simulink model "IEEE9Buses"  (R2024b)
settings: Solver=FixedStepAuto  StartTime=0  StopTime=5  FixedStep=1e-6  RelTol=1e-3
values from neighbouring files (symbols this model uses):
  SG_D_1_D = 0.01056    [SG9_parameters.m]
  SG_D_1_EnableSaturation = 0    [SG9_parameters.m]
  SG_D_1_f0 = 60    [SG9_parameters.m]
  SG_D_1_H = 7.5    [SG9_parameters.m]
  SG_D_1_K_A = 20    [SG9_parameters.m]
  SG_D_1_K_E = 1.000000e+1    (= 10)    [SG9_parameters.m]
  SG_D_1_K_F = 2.363    [SG9_parameters.m]
  SG_D_1_K_s = 5    [SG9_parameters.m]
  SG_D_1_R_a = 0.001088    [SG9_parameters.m]
  SG_D_1_S_A = 1    [SG9_parameters.m]
  SG_D_1_S_B = 0.103    [SG9_parameters.m]
  SG_D_1_S_N = 10.659857    [SG9_parameters.m]
  SG_D_1_SpeedPara = 200    [SG9_parameters.m]
  SG_D_1_T_0 = 0.720173    [SG9_parameters.m]
  SG_D_1_T_1 = 0.3    [SG9_parameters.m]
  SG_D_1_T_2 = 0.05    [SG9_parameters.m]
  SG_D_1_T_3 = 0.02    [SG9_parameters.m]
  SG_D_1_T_4 = 0.005    [SG9_parameters.m]
  SG_D_1_T_A = 0.02    [SG9_parameters.m]
  SG_D_1_T_dd = 8.000000e+0    (= 8)    [SG9_parameters.m]
  SG_D_1_T_ddd = 0.04    [SG9_parameters.m]
  SG_D_1_T_E = 0.314    [SG9_parameters.m]
  SG_D_1_T_F = 0.35    [SG9_parameters.m]
  SG_D_1_T_qd = 0.8    [SG9_parameters.m]
  SG_D_1_T_qdd = 0.02    [SG9_parameters.m]
  SG_D_1_T_speed = 0.1    [SG9_parameters.m]
  SG_D_1_T_w = 0.5    [SG9_parameters.m]
  SG_D_1_V_ref = 1.990276    [SG9_parameters.m]
  SG_D_1_w_ref = 376.991118    [SG9_parameters.m]
  SG_D_1_x_d = 1.9    [SG9_parameters.m]
  SG_D_1_x_dd = 0.302    [SG9_parameters.m]
  SG_D_1_x_ddd = 0.204    [SG9_parameters.m]
  SG_D_1_x_l = 0.05    [SG9_parameters.m]
  SG_D_1_x_q = 1.3    [SG9_parameters.m]
  SG_D_1_x_qd = 0.5    [SG9_parameters.m]
  SG_D_1_x_qdd = 0.3    [SG9_parameters.m]
  SG_D_2_D = 0.01056    [SG9_parameters.m]
  SG_D_2_EnableSaturation = 0    [SG9_parameters.m]
  SG_D_2_f0 = 60    [SG9_parameters.m]
  SG_D_2_H = 7.5    [SG9_parameters.m]
  SG_D_2_K_A = 20    [SG9_parameters.m]
  SG_D_2_K_E = 1.000000e+1    (= 10)    [SG9_parameters.m]
  SG_D_2_K_F = 2.363    [SG9_parameters.m]
  SG_D_2_K_s = 0.5    [SG9_parameters.m]
  SG_D_2_R_a = 0.001088    [SG9_parameters.m]
  SG_D_2_S_A = 1    [SG9_parameters.m]
  SG_D_2_S_B = 0.103    [SG9_parameters.m]
  SG_D_2_S_N = 10.659857    [SG9_parameters.m]
  SG_D_2_SpeedPara = 200    [SG9_parameters.m]
  SG_D_2_T_0 = 1.632913    [SG9_parameters.m]
  SG_D_2_T_1 = 0.2    [SG9_parameters.m]
  SG_D_2_T_2 = 0.05    [SG9_parameters.m]
  SG_D_2_T_3 = 0.02    [SG9_parameters.m]
  SG_D_2_T_4 = 0.005    [SG9_parameters.m]
  SG_D_2_T_A = 0.02    [SG9_parameters.m]
  SG_D_2_T_dd = 8.000000e+0    (= 8)    [SG9_parameters.m]
  SG_D_2_T_ddd = 0.04    [SG9_parameters.m]
  SG_D_2_T_E = 0.314    [SG9_parameters.m]
  SG_D_2_T_F = 0.35    [SG9_parameters.m]
  SG_D_2_T_qd = 0.8    [SG9_parameters.m]
  SG_D_2_T_qdd = 0.02    [SG9_parameters.m]
  SG_D_2_T_speed = 0.1    [SG9_parameters.m]
  SG_D_2_T_w = 0.5    [SG9_parameters.m]
  SG_D_2_V_ref = 2.662631    [SG9_parameters.m]
  SG_D_2_w_ref = 376.991118    [SG9_parameters.m]
  SG_D_2_x_d = 1.9    [SG9_parameters.m]
  SG_D_2_x_dd = 0.302    [SG9_parameters.m]
  SG_D_2_x_ddd = 0.204    [SG9_parameters.m]
  SG_D_2_x_l = 0.05    [SG9_parameters.m]
  SG_D_2_x_q = 1.3    [SG9_parameters.m]
  SG_D_2_x_qd = 0.5    [SG9_parameters.m]
  SG_D_2_x_qdd = 0.3    [SG9_parameters.m]
  SG_D_3_D = 0.01056    [SG9_parameters.m]
  SG_D_3_EnableSaturation = 0    [SG9_parameters.m]
  SG_D_3_f0 = 60    [SG9_parameters.m]
  SG_D_3_H = 7.5    [SG9_parameters.m]
  SG_D_3_K_A = 20    [SG9_parameters.m]
  SG_D_3_K_E = 1.000000e+1    (= 10)    [SG9_parameters.m]
  SG_D_3_K_F = 2.363    [SG9_parameters.m]
  SG_D_3_K_s = 0.5    [SG9_parameters.m]
  SG_D_3_R_a = 0.001088    [SG9_parameters.m]
  SG_D_3_S_A = 1    [SG9_parameters.m]
  SG_D_3_S_B = 0.103    [SG9_parameters.m]
  SG_D_3_S_N = 10.659857    [SG9_parameters.m]
  SG_D_3_SpeedPara = 200    [SG9_parameters.m]
  SG_D_3_T_0 = 0.850788    [SG9_parameters.m]
  SG_D_3_T_1 = 0.2    [SG9_parameters.m]
  SG_D_3_T_2 = 0.05    [SG9_parameters.m]
  SG_D_3_T_3 = 0.02    [SG9_parameters.m]
  SG_D_3_T_4 = 0.005    [SG9_parameters.m]
  SG_D_3_T_A = 0.02    [SG9_parameters.m]
  SG_D_3_T_dd = 8.000000e+0    (= 8)    [SG9_parameters.m]
  SG_D_3_T_ddd = 0.04    [SG9_parameters.m]
  SG_D_3_T_E = 0.314    [SG9_parameters.m]
  SG_D_3_T_F = 0.35    [SG9_parameters.m]
  SG_D_3_T_qd = 0.8    [SG9_parameters.m]
  SG_D_3_T_qdd = 0.02    [SG9_parameters.m]
  SG_D_3_T_speed = 0.1    [SG9_parameters.m]
  SG_D_3_T_w = 0.5    [SG9_parameters.m]
  SG_D_3_V_ref = 1.915682    [SG9_parameters.m]
  SG_D_3_w_ref = 376.991118    [SG9_parameters.m]
  SG_D_3_x_d = 1.9    [SG9_parameters.m]
  SG_D_3_x_dd = 0.302    [SG9_parameters.m]
  SG_D_3_x_ddd = 0.204    [SG9_parameters.m]
  SG_D_3_x_l = 0.05    [SG9_parameters.m]
  SG_D_3_x_q = 1.3    [SG9_parameters.m]
  SG_D_3_x_qd = 0.5    [SG9_parameters.m]
  SG_D_3_x_qdd = 0.3    [SG9_parameters.m]
(part 2 of 9)

== system IEEE9Buses/SG_D_3 ==
  v_d_SG_D_3 : Inport
  v_q_SG_D_3 : Inport  Port=2
  E_fd_SG_D_3 : Integrator  InitialCondition=1.8313641649557557
  Px_1_SG_D_3 : Integrator  InitialCondition=0.0
  Px_2_SG_D_3 : Integrator  InitialCondition=0.0
  Px_3_SG_D_3 : Integrator  InitialCondition=2.300913107602939e-24
  R_f_SG_D_3 : Integrator  InitialCondition=12.364324347972719
  T_e_SG_D_3_block : Subsystem
  T_m_SG_D_3 : Integrator  InitialCondition=0.8507875286404913
  V_f_SG_D_3 : Integrator  InitialCondition=18.313641649557557
  d_E_fd_SG_D_3_block : Subsystem
  d_Px_1_SG_D_3_block : Subsystem
  d_Px_2_SG_D_3_block : Subsystem
  d_Px_3_SG_D_3_block : Subsystem
  d_R_f_SG_D_3_block : Subsystem
  d_T_m_SG_D_3_block : Subsystem
  d_V_f_SG_D_3_block : Subsystem
  d_psi_1d_SG_D_3_block : Subsystem
  d_psi_d_SG_D_3_block : Subsystem
  d_psi_fd_SG_D_3_block : Subsystem
  d_psi_gq_SG_D_3_block : Subsystem
  d_psi_kq_SG_D_3_block : Subsystem
  d_psi_q_SG_D_3_block : Subsystem
  d_theta_SG_D_3_block : Subsystem
  d_w_SG_D_3_block : Subsystem
  i_d_SG_D_3_block : Subsystem
  i_q_SG_D_3_block : Subsystem
  psi_1d_SG_D_3 : Integrator  InitialCondition=0.6849000717806094
  psi_d_SG_D_3 : Integrator  InitialCondition=0.6539145557488486
  psi_fd_SG_D_3 : Integrator  InitialCondition=0.8410670725806834
  psi_gq_SG_D_3 : Integrator  InitialCondition=0.46633252147547377
  psi_kq_SG_D_3 : Integrator  InitialCondition=-0.7286445648054278
  psi_q_SG_D_3 : Integrator  InitialCondition=-0.757790347397645
  theta_SG_D_3 : Integrator  InitialCondition=0.9421581999064681
  theta_SG_D_3_out_block : Subsystem
  w_SG_D_3 : Integrator  InitialCondition=376.99111843077515
  w_SG_D_3_out_block : Subsystem
  i_d_SG_D_3 : Outport
  i_q_SG_D_3 : Outport  Port=2
  T_e_SG_D_3 : Outport  Port=3
  w_SG_D_3_out : Outport  Port=4
  theta_SG_D_3_out : Outport  Port=5
  wires:
  d_Px_1_SG_D_3_block/1(Blockout_d_Px_1_SG_D_3_0a11a) -> Px_1_SG_D_3/1
  w_SG_D_3/1 -> d_psi_d_SG_D_3_block/9(State_w_SG_D_3_3c685), d_w_SG_D_3_block/1(State_w_SG_D_3_2cb2d), d_V_f_SG_D_3_block/13(State_w_SG_D_3_1e0b2), d_V_f_SG_D_3_block/8(State_w_SG_D_3_c925a), d_psi_q_SG_D_3_block/9(State_w_SG_D_3_05eca), d_theta_SG_D_3_block/1(State_w_SG_D_3_9ea4f), d_Px_1_SG_D_3_block/2(State_w_SG_D_3_03ebd), d_Px_2_SG_D_3_block/4(State_w_SG_D_3_8dc04), d_Px_3_SG_D_3_block/6(State_w_SG_D_3_3061a), w_SG_D_3_out_block/1(State_w_SG_D_3_bbd42), d_T_m_SG_D_3_block/1(State_w_SG_D_3_82c70)
  d_Px_2_SG_D_3_block/1(Blockout_d_Px_2_SG_D_3_19155) -> Px_2_SG_D_3/1
  R_f_SG_D_3/1 -> d_V_f_SG_D_3_block/2(State_R_f_SG_D_3_a5ffb), d_R_f_SG_D_3_block/2(State_R_f_SG_D_3_37387)
  w_SG_D_3_out_block/1(Blockout_w_SG_D_3_out_93636) -> w_SG_D_3_out/1
  d_T_m_SG_D_3_block/1(Blockout_d_T_m_SG_D_3_5c1e7) -> T_m_SG_D_3/1
  d_w_SG_D_3_block/1(Blockout_d_w_SG_D_3_8c702) -> w_SG_D_3/1
  Px_1_SG_D_3/1 -> d_Px_3_SG_D_3_block/4(State_Px_1_SG_D_3_747be), d_Px_1_SG_D_3_block/1(State_Px_1_SG_D_3_a2521), d_Px_3_SG_D_3_block/5(State_Px_1_SG_D_3_3120b), d_Px_2_SG_D_3_block/2(State_Px_1_SG_D_3_ddb4e), d_Px_2_SG_D_3_block/3(State_Px_1_SG_D_3_337bf)
  d_theta_SG_D_3_block/1(Blockout_d_theta_SG_D_3_9d209) -> theta_SG_D_3/1
  psi_fd_SG_D_3/1 -> d_psi_fd_SG_D_3_block/4(State_psi_fd_SG_D_3_4a37b), d_psi_fd_SG_D_3_block/7(State_psi_fd_SG_D_3_d3958), d_psi_fd_SG_D_3_block/2(State_psi_fd_SG_D_3_8c274), d_psi_d_SG_D_3_block/3(State_psi_fd_SG_D_3_e8974), d_psi_fd_SG_D_3_block/10(State_psi_fd_SG_D_3_265a7), i_d_SG_D_3_block/7(State_psi_fd_SG_D_3_3705f), d_psi_1d_SG_D_3_block/2(State_psi_fd_SG_D_3_31a8d), i_q_SG_D_3_block/7(State_psi_fd_SG_D_3_e8d39), d_w_SG_D_3_block/10(State_psi_fd_SG_D_3_90538), d_V_f_SG_D_3_block/6(State_psi_fd_SG_D_3_d2e25), T_e_SG_D_3_block/8(State_psi_fd_SG_D_3_cc739), d_psi_1d_SG_D_3_block/5(State_psi_fd_SG_D_3_47081)
  d_Px_3_SG_D_3_block/1(Blockout_d_Px_3_SG_D_3_77867) -> Px_3_SG_D_3/1
  psi_kq_SG_D_3/1 -> d_psi_gq_SG_D_3_block/5(State_psi_kq_SG_D_3_e1997), d_psi_gq_SG_D_3_block/8(State_psi_kq_SG_D_3_4d97e), d_psi_kq_SG_D_3_block/2(State_psi_kq_SG_D_3_9a42a), d_psi_q_SG_D_3_block/2(State_psi_kq_SG_D_3_b8c88), d_psi_kq_SG_D_3_block/4(State_psi_kq_SG_D_3_37576), d_psi_gq_SG_D_3_block/3(State_psi_kq_SG_D_3_22d72), d_V_f_SG_D_3_block/10(State_psi_kq_SG_D_3_1bd63), i_q_SG_D_3_block/2(State_psi_kq_SG_D_3_c33f6), i_d_SG_D_3_block/2(State_psi_kq_SG_D_3_f6fb5), T_e_SG_D_3_block/3(State_psi_kq_SG_D_3_18e1d), d_w_SG_D_3_block/5(State_psi_kq_SG_D_3_8e402)
  psi_d_SG_D_3/1 -> d_psi_fd_SG_D_3_block/6(State_psi_d_SG_D_3_264cd), d_psi_fd_SG_D_3_block/9(State_psi_d_SG_D_3_3305b), d_psi_d_SG_D_3_block/2(State_psi_d_SG_D_3_5cf2c), d_psi_q_SG_D_3_block/8(State_psi_d_SG_D_3_5ea0e), d_psi_1d_SG_D_3_block/4(State_psi_d_SG_D_3_c9b51), d_w_SG_D_3_block/3(State_psi_d_SG_D_3_3eecb), d_V_f_SG_D_3_block/5(State_psi_d_SG_D_3_beaee), d_w_SG_D_3_block/9(State_psi_d_SG_D_3_8d91e), d_V_f_SG_D_3_block/12(State_psi_d_SG_D_3_b0b24), i_q_SG_D_3_block/6(State_psi_d_SG_D_3_d5142), T_e_SG_D_3_block/1(State_psi_d_SG_D_3_17815), i_d_SG_D_3_block/6(State_psi_d_SG_D_3_c47d7), T_e_SG_D_3_block/7(State_psi_d_SG_D_3_9e4e7)
  T_m_SG_D_3/1 -> d_T_m_SG_D_3_block/2(State_T_m_SG_D_3_51fff), d_w_SG_D_3_block/2(State_T_m_SG_D_3_8a11b)
  v_d_SG_D_3/1 -> d_psi_d_SG_D_3_block/4(Input_v_d_SG_D_3_a409b), d_psi_q_SG_D_3_block/4(Input_v_d_SG_D_3_fa4a6)
  v_q_SG_D_3/1 -> d_psi_d_SG_D_3_block/6(Input_v_q_SG_D_3_73a19), d_psi_q_SG_D_3_block/6(Input_v_q_SG_D_3_d1053)
  theta_SG_D_3/1 -> d_psi_d_SG_D_3_block/5(State_theta_SG_D_3_fa0de), d_psi_q_SG_D_3_block/5(State_theta_SG_D_3_c2f12), d_psi_q_SG_D_3_block/7(State_theta_SG_D_3_c1394), i_d_SG_D_3_block/4(State_theta_SG_D_3_f2e5f), d_psi_d_SG_D_3_block/7(State_theta_SG_D_3_450d2), i_d_SG_D_3_block/8(State_theta_SG_D_3_0b124), i_q_SG_D_3_block/4(State_theta_SG_D_3_ac3c7), theta_SG_D_3_out_block/1(State_theta_SG_D_3_cae6d), i_q_SG_D_3_block/8(State_theta_SG_D_3_89a28)
  Px_2_SG_D_3/1 -> d_Px_2_SG_D_3_block/1(State_Px_2_SG_D_3_70e41), d_Px_3_SG_D_3_block/2(State_Px_2_SG_D_3_2a129), d_Px_3_SG_D_3_block/3(State_Px_2_SG_D_3_4e92f)
  psi_gq_SG_D_3/1 -> d_psi_q_SG_D_3_block/1(State_psi_gq_SG_D_3_f88ed), d_psi_gq_SG_D_3_block/1(State_psi_gq_SG_D_3_dcbd7), d_psi_gq_SG_D_3_block/2(State_psi_gq_SG_D_3_25e31), d_psi_gq_SG_D_3_block/4(State_psi_gq_SG_D_3_f44c4), d_w_SG_D_3_block/4(State_psi_gq_SG_D_3_0eb2f), i_d_SG_D_3_block/1(State_psi_gq_SG_D_3_f9205), i_q_SG_D_3_block/1(State_psi_gq_SG_D_3_7b6eb), d_psi_kq_SG_D_3_block/3(State_psi_gq_SG_D_3_70610), T_e_SG_D_3_block/2(State_psi_gq_SG_D_3_9a032), d_V_f_SG_D_3_block/9(State_psi_gq_SG_D_3_ee363), d_psi_kq_SG_D_3_block/1(State_psi_gq_SG_D_3_0b255), d_psi_gq_SG_D_3_block/7(State_psi_gq_SG_D_3_9c664)
  psi_q_SG_D_3/1 -> d_psi_d_SG_D_3_block/8(State_psi_q_SG_D_3_3cdee), d_psi_q_SG_D_3_block/3(State_psi_q_SG_D_3_144cc), d_psi_gq_SG_D_3_block/6(State_psi_q_SG_D_3_5ec2a), d_psi_gq_SG_D_3_block/9(State_psi_q_SG_D_3_66397), d_psi_kq_SG_D_3_block/5(State_psi_q_SG_D_3_7d7d5), i_d_SG_D_3_block/3(State_psi_q_SG_D_3_097ac), d_V_f_SG_D_3_block/11(State_psi_q_SG_D_3_e61a9), d_V_f_SG_D_3_block/7(State_psi_q_SG_D_3_65fee), i_q_SG_D_3_block/3(State_psi_q_SG_D_3_85401), T_e_SG_D_3_block/4(State_psi_q_SG_D_3_3fc53), d_w_SG_D_3_block/7(State_psi_q_SG_D_3_f5035), T_e_SG_D_3_block/5(State_psi_q_SG_D_3_9d696), d_w_SG_D_3_block/6(State_psi_q_SG_D_3_4c6f6)
  d_psi_kq_SG_D_3_block/1(Blockout_d_psi_kq_SG_D_3_b0c25) -> psi_kq_SG_D_3/1
  psi_1d_SG_D_3/1 -> d_psi_fd_SG_D_3_block/3(State_psi_1d_SG_D_3_ced24), d_psi_fd_SG_D_3_block/5(State_psi_1d_SG_D_3_58f7d), d_psi_fd_SG_D_3_block/8(State_psi_1d_SG_D_3_6cc6d), d_psi_d_SG_D_3_block/1(State_psi_1d_SG_D_3_df20d), d_psi_1d_SG_D_3_block/1(State_psi_1d_SG_D_3_400ff), d_V_f_SG_D_3_block/4(State_psi_1d_SG_D_3_5da7b), d_psi_1d_SG_D_3_block/3(State_psi_1d_SG_D_3_f2eaa), d_w_SG_D_3_block/8(State_psi_1d_SG_D_3_a0e82), i_d_SG_D_3_block/5(State_psi_1d_SG_D_3_3346a), i_q_SG_D_3_block/5(State_psi_1d_SG_D_3_c21a4), T_e_SG_D_3_block/6(State_psi_1d_SG_D_3_e0c74)
  d_psi_q_SG_D_3_block/1(Blockout_d_psi_q_SG_D_3_07f24) -> psi_q_SG_D_3/1
  d_R_f_SG_D_3_block/1(Blockout_d_R_f_SG_D_3_9bb7b) -> R_f_SG_D_3/1
  theta_SG_D_3_out_block/1(Blockout_theta_SG_D_3_out_1963e) -> theta_SG_D_3_out/1
  d_V_f_SG_D_3_block/1(Blockout_d_V_f_SG_D_3_f5fd7) -> V_f_SG_D_3/1
  T_e_SG_D_3_block/1(Blockout_T_e_SG_D_3_2b576) -> T_e_SG_D_3/1
  d_psi_gq_SG_D_3_block/1(Blockout_d_psi_gq_SG_D_3_5f8a8) -> psi_gq_SG_D_3/1
  i_d_SG_D_3_block/1(Blockout_i_d_SG_D_3_0f9ed) -> i_d_SG_D_3/1
  d_psi_d_SG_D_3_block/1(Blockout_d_psi_d_SG_D_3_6cd1a) -> psi_d_SG_D_3/1
  d_psi_1d_SG_D_3_block/1(Blockout_d_psi_1d_SG_D_3_883d4) -> psi_1d_SG_D_3/1
  i_q_SG_D_3_block/1(Blockout_i_q_SG_D_3_01fe5) -> i_q_SG_D_3/1
  V_f_SG_D_3/1 -> d_V_f_SG_D_3_block/14(State_V_f_SG_D_3_da029), d_E_fd_SG_D_3_block/2(State_V_f_SG_D_3_25ca2)
  Px_3_SG_D_3/1 -> d_V_f_SG_D_3_block/3(State_Px_3_SG_D_3_ea3e2), d_Px_3_SG_D_3_block/1(State_Px_3_SG_D_3_d10c2)
  d_E_fd_SG_D_3_block/1(Blockout_d_E_fd_SG_D_3_8d01f) -> E_fd_SG_D_3/1
  E_fd_SG_D_3/1 -> d_V_f_SG_D_3_block/1(State_E_fd_SG_D_3_5b543), d_R_f_SG_D_3_block/1(State_E_fd_SG_D_3_87a80), d_E_fd_SG_D_3_block/1(State_E_fd_SG_D_3_1d006), d_psi_fd_SG_D_3_block/1(State_E_fd_SG_D_3_2d5b6)
  d_psi_fd_SG_D_3_block/1(Blockout_d_psi_fd_SG_D_3_c1dbd) -> psi_fd_SG_D_3/1

== system IEEE9Buses/AC_1/d_id_line_1_4_block ==
  note: d_id_line_1_4 in SG9
      | $376.991118430775\,\mathrm{iq}_{\mathrm{line},1,4}+6544.98469497874\,\mathrm{vd}_{\mathrm{bus},1}-6544.98469497874\,\mathrm{vd}_{\mathrm{bus},4}$
      | Automatically generated on 2025-09-12 21:34:30 .
  State_iq_line_1_4_a5e26 : Inport
  State_vd_bus_1_adf11 : Inport  Port=2
  State_vd_bus_4_44d4f : Inport  Port=3
  Add_12319 : Sum
  Constant_376.991118430775_fd345 : Constant  Value=376.991118430775
  Constant_6544.98469497874_78b0a : Constant  Value=6544.98469497874
  Constant_6544.98469497874_aadf5 : Constant  Value=6544.98469497874
  Product_b0358 : Product
  Product_ba79a : Product
  Product_f9389 : Product
  Subtract_2baca : Sum  Inputs=+-
  Blockout_d_id_line_1_4_93c8d : Outport
  wires:
  Constant_376.991118430775_fd345/1 -> Product_ba79a/1
  Product_f9389/1 -> Add_12319/2
  State_iq_line_1_4_a5e26/1 -> Product_ba79a/2
  Subtract_2baca/1 -> Blockout_d_id_line_1_4_93c8d/1
  Constant_6544.98469497874_78b0a/1 -> Product_f9389/1
  Product_ba79a/1 -> Add_12319/1
  State_vd_bus_1_adf11/1 -> Product_f9389/2
  Constant_6544.98469497874_aadf5/1 -> Product_b0358/1
  State_vd_bus_4_44d4f/1 -> Product_b0358/2
  Add_12319/1 -> Subtract_2baca/1
  Product_b0358/1 -> Subtract_2baca/2

== system IEEE9Buses/AC_1/d_id_line_3_6_block ==
  note: d_id_line_3_6 in SG9
      | $376.991118430775\,\mathrm{iq}_{\mathrm{line},3,6}+6433.29553636135\,\mathrm{vd}_{\mathrm{bus},3}-6433.29553636135\,\mathrm{vd}_{\mathrm{bus},6}$
      | Automatically generated on 2025-09-12 21:34:37 .
  State_iq_line_3_6_282d0 : Inport
  State_vd_bus_3_4df94 : Inport  Port=2
  State_vd_bus_6_a239d : Inport  Port=3
  Add_ee434 : Sum
  Constant_376.991118430775_70988 : Constant  Value=376.991118430775
  Constant_6433.29553636135_43692 : Constant  Value=6433.29553636135
  Constant_6433.29553636135_b371c : Constant  Value=6433.29553636135
  Product_4a8bb : Product
  Product_8bfb3 : Product
  Product_e0a87 : Product
  Subtract_2a009 : Sum  Inputs=+-
  Blockout_d_id_line_3_6_e09c3 : Outport
  wires:
  State_vd_bus_3_4df94/1 -> Product_8bfb3/2
  Constant_376.991118430775_70988/1 -> Product_e0a87/1
  Product_8bfb3/1 -> Add_ee434/2
  State_iq_line_3_6_282d0/1 -> Product_e0a87/2
  Constant_6433.29553636135_43692/1 -> Product_8bfb3/1
  Product_e0a87/1 -> Add_ee434/1
  Constant_6433.29553636135_b371c/1 -> Product_4a8bb/1
  State_vd_bus_6_a239d/1 -> Product_4a8bb/2
  Add_ee434/1 -> Subtract_2a009/1
  Product_4a8bb/1 -> Subtract_2a009/2
  Subtract_2a009/1 -> Blockout_d_id_line_3_6_e09c3/1

== system IEEE9Buses/AC_1/d_id_line_4_5_block ==
  note: d_id_line_4_5 in SG9
      | $376.991118430775\,\mathrm{iq}_{\mathrm{line},4,5}-69.6614023187302\,\mathrm{id}_{\mathrm{line},4,5}+4097.7295481606\,\mathrm{vd}_{\mathrm{bus},4}-4097.7295481606\,\mathrm{vd}_{\mathrm{bus},5}$
      | Automatically generated on 2025-09-12 21:34:32 .
  State_id_line_4_5_9d9bf : Inport
  State_iq_line_4_5_254e7 : Inport  Port=2
  State_vd_bus_4_779cd : Inport  Port=3
  State_vd_bus_5_5d0f4 : Inport  Port=4
  Add_06947 : Sum
  Add_44019 : Sum
  Constant_-69.6614023187302_e72f9 : Constant  Value=-69.6614023187302
  Constant_376.991118430775_9d07c : Constant  Value=376.991118430775
  Constant_4097.7295481606_1efbc : Constant  Value=4097.7295481606
  Constant_4097.7295481606_ceea8 : Constant  Value=4097.7295481606
  Product_0dc6c : Product
  Product_835b4 : Product
  Product_85d7f : Product
  Product_ceabb : Product
  Subtract_2702d : Sum  Inputs=+-
  Blockout_d_id_line_4_5_01c13 : Outport
  wires:
  Constant_-69.6614023187302_e72f9/1 -> Product_0dc6c/1
  Product_85d7f/1 -> Add_06947/2
  State_id_line_4_5_9d9bf/1 -> Product_0dc6c/2
  Constant_376.991118430775_9d07c/1 -> Product_85d7f/1
  State_iq_line_4_5_254e7/1 -> Product_85d7f/2
  Product_0dc6c/1 -> Add_06947/1
  Constant_4097.7295481606_1efbc/1 -> Product_ceabb/1
  State_vd_bus_4_779cd/1 -> Product_ceabb/2
  Add_06947/1 -> Add_44019/1
  Product_ceabb/1 -> Add_44019/2
  Constant_4097.7295481606_ceea8/1 -> Product_835b4/1
  State_vd_bus_5_5d0f4/1 -> Product_835b4/2
  Add_44019/1 -> Subtract_2702d/1
  Product_835b4/1 -> Subtract_2702d/2
  Subtract_2702d/1 -> Blockout_d_id_line_4_5_01c13/1

== system IEEE9Buses/AC_1/d_id_line_5_6_block ==
  note: d_id_line_5_6 in SG9
      | $376.991118430775\,\mathrm{iq}_{\mathrm{line},5,6}-86.4861977576484\,\mathrm{id}_{\mathrm{line},5,6}+2217.59481429868\,\mathrm{vd}_{\mathrm{bus},5}-2217.59481429868\,\mathrm{vd}_{\mathrm{bus},6}$
      | Automatically generated on 2025-09-12 21:34:35 .
  State_id_line_5_6_30ca9 : Inport
  State_iq_line_5_6_587be : Inport  Port=2
  State_vd_bus_5_135fa : Inport  Port=3
  State_vd_bus_6_469ee : Inport  Port=4
  Add_737bf : Sum
  Add_d0fe5 : Sum
  Constant_-86.4861977576484_ae60e : Constant  Value=-86.4861977576484
  Constant_2217.59481429868_8308b : Constant  Value=2217.59481429868
  Constant_2217.59481429868_be8db : Constant  Value=2217.59481429868
  Constant_376.991118430775_bc4c5 : Constant  Value=376.991118430775
  Product_10b3d : Product
  Product_6682f : Product
  Product_828c4 : Product
  Product_df755 : Product
  Subtract_25241 : Sum  Inputs=+-
  Blockout_d_id_line_5_6_0d6a1 : Outport
  wires:
  Constant_-86.4861977576484_ae60e/1 -> Product_828c4/1
  Product_df755/1 -> Add_d0fe5/2
  State_id_line_5_6_30ca9/1 -> Product_828c4/2
  Constant_376.991118430775_bc4c5/1 -> Product_df755/1
  Product_828c4/1 -> Add_d0fe5/1
  State_iq_line_5_6_587be/1 -> Product_df755/2
  Constant_2217.59481429868_8308b/1 -> Product_10b3d/1
  Product_6682f/1 -> Subtract_25241/2
  State_vd_bus_5_135fa/1 -> Product_10b3d/2
  Add_d0fe5/1 -> Add_737bf/1
  Product_10b3d/1 -> Add_737bf/2
  Constant_2217.59481429868_be8db/1 -> Product_6682f/1
  State_vd_bus_6_469ee/1 -> Product_6682f/2
  Add_737bf/1 -> Subtract_25241/1
  Subtract_25241/1 -> Blockout_d_id_line_5_6_0d6a1/1

== system IEEE9Buses/AC_1/d_id_line_6_7_block ==
  note: d_id_line_6_7 in SG9
      | $376.991118430775\,\mathrm{iq}_{\mathrm{line},6,7}-44.5058959258554\,\mathrm{id}_{\mathrm{line},6,7}+3739.99125427356\,\mathrm{vd}_{\mathrm{bus},6}-3739.99125427356\,\mathrm{vd}_{\mathrm{bus},7}$
      | Automatically generated on 2025-09-12 21:34:39 .
  State_id_line_6_7_a6336 : Inport
  State_iq_line_6_7_95ec9 : Inport  Port=2
  State_vd_bus_6_443fc : Inport  Port=3
  State_vd_bus_7_82461 : Inport  Port=4
  Add_35f00 : Sum
  Add_ad8cf : Sum
  Constant_-44.5058959258554_cb7d9 : Constant  Value=-44.5058959258554
  Constant_3739.99125427356_2a8da : Constant  Value=3739.99125427356
  Constant_3739.99125427356_6b808 : Constant  Value=3739.99125427356
  Constant_376.991118430775_61819 : Constant  Value=376.991118430775
  Product_345ed : Product
  Product_a947a : Product
  Product_e0946 : Product
  Product_fa4d0 : Product
  Subtract_111b2 : Sum  Inputs=+-
  Blockout_d_id_line_6_7_75140 : Outport
  wires:
  Constant_-44.5058959258554_cb7d9/1 -> Product_345ed/1
  Product_fa4d0/1 -> Add_35f00/2
  State_id_line_6_7_a6336/1 -> Product_345ed/2
  Constant_376.991118430775_61819/1 -> Product_fa4d0/1
  State_iq_line_6_7_95ec9/1 -> Product_fa4d0/2
  Product_345ed/1 -> Add_35f00/1
  Constant_3739.99125427356_6b808/1 -> Product_a947a/1
  State_vd_bus_6_443fc/1 -> Product_a947a/2
  Add_35f00/1 -> Add_ad8cf/1
  Product_a947a/1 -> Add_ad8cf/2
  Constant_3739.99125427356_2a8da/1 -> Product_e0946/1
  State_vd_bus_7_82461/1 -> Product_e0946/2
  Add_ad8cf/1 -> Subtract_111b2/1
  Product_e0946/1 -> Subtract_111b2/2
  Subtract_111b2/1 -> Blockout_d_id_line_6_7_75140/1

== system IEEE9Buses/AC_1/d_id_line_7_8_block ==
  note: d_id_line_7_8 in SG9
      | $376.991118430775\,\mathrm{iq}_{\mathrm{line},7,8}-44.5058959258554\,\mathrm{id}_{\mathrm{line},7,8}+5235.98775598299\,\mathrm{vd}_{\mathrm{bus},7}-5235.98775598299\,\mathrm{vd}_{\mathrm{bus},8}$
      | Automatically generated on 2025-09-12 21:34:41 .
  State_id_line_7_8_3b707 : Inport
  State_iq_line_7_8_ca362 : Inport  Port=2
  State_vd_bus_7_ec582 : Inport  Port=3
  State_vd_bus_8_932d1 : Inport  Port=4
  Add_1c9b9 : Sum
  Add_dfa35 : Sum
  Constant_-44.5058959258554_7f097 : Constant  Value=-44.5058959258554
  Constant_376.991118430775_9e6c3 : Constant  Value=376.991118430775
  Constant_5235.98775598299_0b6b0 : Constant  Value=5235.98775598299
  Constant_5235.98775598299_c1a6d : Constant  Value=5235.98775598299
  Product_3f519 : Product
  Product_cb839 : Product
  Product_cd3f9 : Product
  Product_f6bcc : Product
  Subtract_1072e : Sum  Inputs=+-
  Blockout_d_id_line_7_8_9746d : Outport
  wires:
  Constant_-44.5058959258554_7f097/1 -> Product_3f519/1
  Product_cd3f9/1 -> Add_dfa35/2
  State_id_line_7_8_3b707/1 -> Product_3f519/2
  Constant_376.991118430775_9e6c3/1 -> Product_cd3f9/1
  Product_3f519/1 -> Add_dfa35/1
  State_iq_line_7_8_ca362/1 -> Product_cd3f9/2
  Constant_5235.98775598299_c1a6d/1 -> Product_f6bcc/1
  State_vd_bus_7_ec582/1 -> Product_f6bcc/2
  Add_dfa35/1 -> Add_1c9b9/1
  Product_f6bcc/1 -> Add_1c9b9/2
  Constant_5235.98775598299_0b6b0/1 -> Product_cb839/1
  State_vd_bus_8_932d1/1 -> Product_cb839/2
  Add_1c9b9/1 -> Subtract_1072e/1
  Product_cb839/1 -> Subtract_1072e/2
  Subtract_1072e/1 -> Blockout_d_id_line_7_8_9746d/1

== system IEEE9Buses/AC_1/d_id_line_8_2_block ==
  note: d_id_line_8_2 in SG9
      | $376.991118430775\,\mathrm{iq}_{\mathrm{line},8,2}-6031.8578948924\,\mathrm{vd}_{\mathrm{bus},2}+6031.8578948924\,\mathrm{vd}_{\mathrm{bus},8}$
      | Automatically generated on 2025-09-12 21:34:43 .
  State_iq_line_8_2_d048e : Inport
  State_vd_bus_2_bbfdf : Inport  Port=2
  State_vd_bus_8_4faee : Inport  Port=3
  Add_80bdd : Sum
  Constant_376.991118430775_c6d43 : Constant  Value=376.991118430775
  Constant_6031.8578948924_aa122 : Constant  Value=6031.8578948924
  Constant_6031.8578948924_f748a : Constant  Value=6031.8578948924
  Product_1c21e : Product
  Product_9571a : Product
  Product_e6e9c : Product
  Subtract_bc58f : Sum  Inputs=+-
  Blockout_d_id_line_8_2_17ce9 : Outport
  wires:
  State_vd_bus_2_bbfdf/1 -> Product_e6e9c/2
  Constant_376.991118430775_c6d43/1 -> Product_9571a/1
  Product_e6e9c/1 -> Subtract_bc58f/2
  State_iq_line_8_2_d048e/1 -> Product_9571a/2
  Constant_6031.8578948924_f748a/1 -> Product_e6e9c/1
  Product_9571a/1 -> Subtract_bc58f/1
  Constant_6031.8578948924_aa122/1 -> Product_1c21e/1
  State_vd_bus_8_4faee/1 -> Product_1c21e/2
  Subtract_bc58f/1 -> Add_80bdd/1
  Product_1c21e/1 -> Add_80bdd/2
  Add_80bdd/1 -> Blockout_d_id_line_8_2_17ce9/1

== system IEEE9Buses/AC_1/d_id_line_8_9_block ==
  note: d_id_line_8_9 in SG9
      | $376.991118430775\,\mathrm{iq}_{\mathrm{line},8,9}-74.9299117377938\,\mathrm{id}_{\mathrm{line},8,9}+2341.55974180606\,\mathrm{vd}_{\mathrm{bus},8}-2341.55974180606\,\mathrm{vd}_{\mathrm{bus},9}$
      | Automatically generated on 2025-09-12 21:34:45 .
  State_id_line_8_9_b15e6 : Inport
  State_iq_line_8_9_9c429 : Inport  Port=2
  State_vd_bus_8_2da45 : Inport  Port=3
  State_vd_bus_9_bcf84 : Inport  Port=4
  Add_1a5dc : Sum
  Add_2b9a6 : Sum
  Constant_-74.9299117377938_e83f7 : Constant  Value=-74.9299117377938
  Constant_2341.55974180606_84f68 : Constant  Value=2341.55974180606
  Constant_2341.55974180606_8c83c : Constant  Value=2341.55974180606
  Constant_376.991118430775_c9a6d : Constant  Value=376.991118430775
  Product_a3c9e : Product
  Product_a4088 : Product
  Product_a59e3 : Product
  Product_a7ced : Product
  Subtract_fa2bb : Sum  Inputs=+-
  Blockout_d_id_line_8_9_50e3a : Outport
  wires:
  Constant_-74.9299117377938_e83f7/1 -> Product_a4088/1
  Product_a3c9e/1 -> Add_1a5dc/2
  State_id_line_8_9_b15e6/1 -> Product_a4088/2
  Constant_376.991118430775_c9a6d/1 -> Product_a3c9e/1
  State_iq_line_8_9_9c429/1 -> Product_a3c9e/2
  Product_a4088/1 -> Add_1a5dc/1
  Constant_2341.55974180606_8c83c/1 -> Product_a7ced/1
  State_vd_bus_8_2da45/1 -> Product_a7ced/2
  Add_1a5dc/1 -> Add_2b9a6/1
  Product_a7ced/1 -> Add_2b9a6/2
  Constant_2341.55974180606_84f68/1 -> Product_a59e3/1
  State_vd_bus_9_bcf84/1 -> Product_a59e3/2
  Add_2b9a6/1 -> Subtract_fa2bb/1
  Product_a59e3/1 -> Subtract_fa2bb/2
  Subtract_fa2bb/1 -> Blockout_d_id_line_8_9_50e3a/1

== system IEEE9Buses/AC_1/d_id_line_9_4_block ==
  note: d_id_line_9_4 in SG9
      | $376.991118430775\,\mathrm{iq}_{\mathrm{line},9,4}-44.3518962859735\,\mathrm{id}_{\mathrm{line},9,4}-4435.18962859735\,\mathrm{vd}_{\mathrm{bus},4}+4435.18962859735\,\mathrm{vd}_{\mathrm{bus},9}$
      | Automatically generated on 2025-09-12 21:34:47 .
  State_id_line_9_4_75390 : Inport
  State_iq_line_9_4_9b423 : Inport  Port=2
  State_vd_bus_4_e2c56 : Inport  Port=3
  State_vd_bus_9_f9bbb : Inport  Port=4
  Add_0d9c2 : Sum
  Add_f584b : Sum
  Constant_-44.3518962859735_35e1f : Constant  Value=-44.3518962859735
  Constant_376.991118430775_11eee : Constant  Value=376.991118430775
  Constant_4435.18962859735_a5be0 : Constant  Value=4435.18962859735
  Constant_4435.18962859735_c4b75 : Constant  Value=4435.18962859735
  Product_b0e4f : Product
  Product_d6df1 : Product
  Product_debda : Product
  Product_e872e : Product
  Subtract_b8ab1 : Sum  Inputs=+-
  Blockout_d_id_line_9_4_bcdf8 : Outport
  wires:
  Constant_-44.3518962859735_35e1f/1 -> Product_e872e/1
  Product_b0e4f/1 -> Add_0d9c2/2
  State_id_line_9_4_75390/1 -> Product_e872e/2
  Constant_376.991118430775_11eee/1 -> Product_b0e4f/1
  Product_e872e/1 -> Add_0d9c2/1
  State_iq_line_9_4_9b423/1 -> Product_b0e4f/2
  Constant_4435.18962859735_c4b75/1 -> Product_d6df1/1
  State_vd_bus_4_e2c56/1 -> Product_d6df1/2
  Add_0d9c2/1 -> Subtract_b8ab1/1
  Product_d6df1/1 -> Subtract_b8ab1/2
  Constant_4435.18962859735_a5be0/1 -> Product_debda/1
  Subtract_b8ab1/1 -> Add_f584b/1
  State_vd_bus_9_f9bbb/1 -> Product_debda/2
  Product_debda/1 -> Add_f584b/2
  Add_f584b/1 -> Blockout_d_id_line_9_4_bcdf8/1

== system IEEE9Buses/AC_1/d_id_load_5_block ==
  note: d_id_load_5 in SG9
      | $376.991118430775\,\mathrm{iq}_{\mathrm{load},5}-1130.97335529233\,\mathrm{id}_{\mathrm{load},5}+1188.5640696821\,\mathrm{vd}_{\mathrm{bus},5}$
      | Automatically generated on 2025-09-12 21:34:25 .
  State_id_load_5_6942d : Inport
  State_iq_load_5_374bd : Inport  Port=2
  State_vd_bus_5_7ebb7 : Inport  Port=3
  Add_8dc55 : Sum
  Add_f6448 : Sum
  Constant_-1130.97335529233_05366 : Constant  Value=-1130.97335529233
  Constant_1188.5640696821_38457 : Constant  Value=1188.5640696821
  Constant_376.991118430775_7034b : Constant  Value=376.991118430775
  Product_52302 : Product
  Product_6ab51 : Product
  Product_7fa7a : Product
  Blockout_d_id_load_5_1877c : Outport
  wires:
  Constant_-1130.97335529233_05366/1 -> Product_7fa7a/1
  Product_52302/1 -> Add_f6448/2
  State_id_load_5_6942d/1 -> Product_7fa7a/2
  Constant_376.991118430775_7034b/1 -> Product_52302/1
  Product_6ab51/1 -> Add_8dc55/2
  State_iq_load_5_374bd/1 -> Product_52302/2
  Product_7fa7a/1 -> Add_f6448/1
  Constant_1188.5640696821_38457/1 -> Product_6ab51/1
  State_vd_bus_5_7ebb7/1 -> Product_6ab51/2
  Add_f6448/1 -> Add_8dc55/1
  Add_8dc55/1 -> Blockout_d_id_load_5_1877c/1

== system IEEE9Buses/AC_1/d_id_load_7_block ==
  note: d_id_load_7 in SG9
      | $376.991118430775\,\mathrm{iq}_{\mathrm{load},7}-1077.11748123079\,\mathrm{id}_{\mathrm{load},7}+1244.53892235533\,\mathrm{vd}_{\mathrm{bus},7}$
      | Automatically generated on 2025-09-12 21:34:27 .
  State_id_load_7_9c11f : Inport
  State_iq_load_7_51219 : Inport  Port=2
  State_vd_bus_7_a9ee9 : Inport  Port=3
  Add_533fc : Sum
  Add_cc379 : Sum
  Constant_-1077.11748123079_c5a3f : Constant  Value=-1077.11748123079
  Constant_1244.53892235533_83ba7 : Constant  Value=1244.53892235533
  Constant_376.991118430775_cf991 : Constant  Value=376.991118430775
  Product_7de1a : Product
  Product_cd34e : Product
  Product_dd6d8 : Product
  Blockout_d_id_load_7_5535f : Outport
  wires:
  Constant_-1077.11748123079_c5a3f/1 -> Product_cd34e/1
  Product_dd6d8/1 -> Add_cc379/2
  State_id_load_7_9c11f/1 -> Product_cd34e/2
  Constant_376.991118430775_cf991/1 -> Product_dd6d8/1
  Product_cd34e/1 -> Add_cc379/1
  State_iq_load_7_51219/1 -> Product_dd6d8/2
  Constant_1244.53892235533_83ba7/1 -> Product_7de1a/1
  State_vd_bus_7_a9ee9/1 -> Product_7de1a/2
  Add_cc379/1 -> Add_533fc/1
  Product_7de1a/1 -> Add_533fc/2
  Add_533fc/1 -> Blockout_d_id_load_7_5535f/1

== system IEEE9Buses/AC_1/d_id_load_9_block ==
  note: d_id_load_9 in SG9
      | $376.991118430775\,\mathrm{iq}_{\mathrm{load},9}-942.477796076938\,\mathrm{id}_{\mathrm{load},9}+1490.22474585066\,\mathrm{vd}_{\mathrm{bus},9}$
      | Automatically generated on 2025-09-12 21:34:28 .
  State_id_load_9_f793a : Inport
  State_iq_load_9_20a57 : Inport  Port=2
  State_vd_bus_9_d8fb5 : Inport  Port=3
  Add_50aed : Sum
  Add_bf7f5 : Sum
  Constant_-942.477796076938_4ddad : Constant  Value=-942.477796076938
  Constant_1490.22474585066_a65d3 : Constant  Value=1490.22474585066
  Constant_376.991118430775_d89bc : Constant  Value=376.991118430775
  Product_3c0f0 : Product
  Product_4bfd4 : Product
  Product_83a02 : Product
  Blockout_d_id_load_9_d90d0 : Outport
  wires:
  Constant_-942.477796076938_4ddad/1 -> Product_83a02/1
  Product_3c0f0/1 -> Add_bf7f5/2
  State_id_load_9_f793a/1 -> Product_83a02/2
  Constant_376.991118430775_d89bc/1 -> Product_3c0f0/1
  Product_83a02/1 -> Add_bf7f5/1
  State_iq_load_9_20a57/1 -> Product_3c0f0/2
  Constant_1490.22474585066_a65d3/1 -> Product_4bfd4/1
  State_vd_bus_9_d8fb5/1 -> Product_4bfd4/2
  Add_bf7f5/1 -> Add_50aed/1
  Product_4bfd4/1 -> Add_50aed/2
  Add_50aed/1 -> Blockout_d_id_load_9_d90d0/1

== system IEEE9Buses/AC_1/d_iq_line_1_4_block ==
  note: d_iq_line_1_4 in SG9
      | $6544.98469497874\,\mathrm{vq}_{\mathrm{bus},1}-376.991118430775\,\mathrm{id}_{\mathrm{line},1,4}-6544.98469497874\,\mathrm{vq}_{\mathrm{bus},4}$
      | Automatically generated on 2025-09-12 21:34:31 .
  State_id_line_1_4_57d80 : Inport
  State_vq_bus_1_b7ee6 : Inport  Port=2
  State_vq_bus_4_b5984 : Inport  Port=3
  Add_35c80 : Sum
  Constant_-376.991118430775_f855d : Constant  Value=-376.991118430775
  Constant_6544.98469497874_a0a5b : Constant  Value=6544.98469497874
  Constant_6544.98469497874_ba131 : Constant  Value=6544.98469497874
  Product_83029 : Product
  Product_dcb40 : Product
  Product_f06cf : Product
  Subtract_1a6d1 : Sum  Inputs=+-
  Blockout_d_iq_line_1_4_afc5f : Outport
  wires:
  Constant_-376.991118430775_f855d/1 -> Product_83029/1
  Product_f06cf/1 -> Add_35c80/2
  State_id_line_1_4_57d80/1 -> Product_83029/2
  Constant_6544.98469497874_a0a5b/1 -> Product_f06cf/1
  Product_83029/1 -> Add_35c80/1
  Subtract_1a6d1/1 -> Blockout_d_iq_line_1_4_afc5f/1
  State_vq_bus_1_b7ee6/1 -> Product_f06cf/2
  Constant_6544.98469497874_ba131/1 -> Product_dcb40/1
  State_vq_bus_4_b5984/1 -> Product_dcb40/2
  Add_35c80/1 -> Subtract_1a6d1/1
  Product_dcb40/1 -> Subtract_1a6d1/2

== system IEEE9Buses/AC_1/d_iq_line_3_6_block ==
  note: d_iq_line_3_6 in SG9
      | $6433.29553636135\,\mathrm{vq}_{\mathrm{bus},3}-376.991118430775\,\mathrm{id}_{\mathrm{line},3,6}-6433.29553636135\,\mathrm{vq}_{\mathrm{bus},6}$
      | Automatically generated on 2025-09-12 21:34:38 .
  State_id_line_3_6_232a9 : Inport
  State_vq_bus_3_b412d : Inport  Port=2
  State_vq_bus_6_14cd6 : Inport  Port=3
  Add_30752 : Sum
  Constant_-376.991118430775_7c554 : Constant  Value=-376.991118430775
  Constant_6433.29553636135_3e254 : Constant  Value=6433.29553636135
  Constant_6433.29553636135_bcb2a : Constant  Value=6433.29553636135
  Product_32f36 : Product
  Product_6e362 : Product
  Product_7dbcc : Product
  Subtract_86ead : Sum  Inputs=+-
  Blockout_d_iq_line_3_6_9df33 : Outport
  wires:
  Constant_-376.991118430775_7c554/1 -> Product_7dbcc/1
  Product_6e362/1 -> Add_30752/2
  State_id_line_3_6_232a9/1 -> Product_7dbcc/2
  Constant_6433.29553636135_3e254/1 -> Product_6e362/1
  Product_7dbcc/1 -> Add_30752/1
  State_vq_bus_3_b412d/1 -> Product_6e362/2
  Constant_6433.29553636135_bcb2a/1 -> Product_32f36/1
  State_vq_bus_6_14cd6/1 -> Product_32f36/2
  Add_30752/1 -> Subtract_86ead/1
  Product_32f36/1 -> Subtract_86ead/2
  Subtract_86ead/1 -> Blockout_d_iq_line_3_6_9df33/1

== system IEEE9Buses/AC_1/d_iq_line_4_5_block ==
  note: d_iq_line_4_5 in SG9
      | $4097.7295481606\,\mathrm{vq}_{\mathrm{bus},4}-69.6614023187302\,\mathrm{iq}_{\mathrm{line},4,5}-376.991118430775\,\mathrm{id}_{\mathrm{line},4,5}-4097.7295481606\,\mathrm{vq}_{\mathrm{bus},5}$
      | Automatically generated on 2025-09-12 21:34:33 .
  State_id_line_4_5_bb2d8 : Inport
  State_iq_line_4_5_78e2b : Inport  Port=2
  State_vq_bus_4_a5b76 : Inport  Port=3
  State_vq_bus_5_6d109 : Inport  Port=4
  Add_e8b5a : Sum
  Constant_-376.991118430775_fce92 : Constant  Value=-376.991118430775
  Constant_4097.7295481606_5305e : Constant  Value=4097.7295481606
  Constant_4097.7295481606_5b98a : Constant  Value=4097.7295481606
  Constant_69.6614023187302_ad837 : Constant  Value=69.6614023187302
  Product_82f1b : Product
  Product_afccc : Product
  Product_b148f : Product
  Product_b2475 : Product
  Subtract_2a1c3 : Sum  Inputs=+-
  Subtract_fd4db : Sum  Inputs=+-
  Blockout_d_iq_line_4_5_7f0d8 : Outport
  wires:
  Constant_-376.991118430775_fce92/1 -> Product_b2475/1
  Constant_69.6614023187302_ad837/1 -> Product_b148f/1
  State_id_line_4_5_bb2d8/1 -> Product_b2475/2
  State_iq_line_4_5_78e2b/1 -> Product_b148f/2
  Product_b2475/1 -> Subtract_2a1c3/1
  Constant_4097.7295481606_5b98a/1 -> Product_82f1b/1
  Product_b148f/1 -> Subtract_2a1c3/2
  State_vq_bus_4_a5b76/1 -> Product_82f1b/2
  Subtract_2a1c3/1 -> Add_e8b5a/1
  Product_82f1b/1 -> Add_e8b5a/2
  Constant_4097.7295481606_5305e/1 -> Product_afccc/1
  State_vq_bus_5_6d109/1 -> Product_afccc/2
  Add_e8b5a/1 -> Subtract_fd4db/1
  Product_afccc/1 -> Subtract_fd4db/2
  Subtract_fd4db/1 -> Blockout_d_iq_line_4_5_7f0d8/1

== system IEEE9Buses/AC_1/d_iq_line_5_6_block ==
  note: d_iq_line_5_6 in SG9
      | $2217.59481429868\,\mathrm{vq}_{\mathrm{bus},5}-86.4861977576484\,\mathrm{iq}_{\mathrm{line},5,6}-376.991118430775\,\mathrm{id}_{\mathrm{line},5,6}-2217.59481429868\,\mathrm{vq}_{\mathrm{bus},6}$
      | Automatically generated on 2025-09-12 21:34:36 .
  State_id_line_5_6_bb5d1 : Inport
  State_iq_line_5_6_03d26 : Inport  Port=2
  State_vq_bus_5_5a835 : Inport  Port=3
  State_vq_bus_6_e6417 : Inport  Port=4
  Add_0d293 : Sum
  Constant_-376.991118430775_ca6b1 : Constant  Value=-376.991118430775
  Constant_2217.59481429868_1f2a1 : Constant  Value=2217.59481429868
  Constant_2217.59481429868_393ef : Constant  Value=2217.59481429868
  Constant_86.4861977576484_5e15a : Constant  Value=86.4861977576484
  Product_4d4ad : Product
  Product_584f5 : Product
  Product_7a064 : Product
  Product_e5a10 : Product
  Subtract_6c7cf : Sum  Inputs=+-
  Subtract_f6ff4 : Sum  Inputs=+-
  Blockout_d_iq_line_5_6_f65e1 : Outport
  wires:
  Constant_-376.991118430775_ca6b1/1 -> Product_7a064/1
  Constant_86.4861977576484_5e15a/1 -> Product_4d4ad/1
  Subtract_6c7cf/1 -> Blockout_d_iq_line_5_6_f65e1/1
  State_id_line_5_6_bb5d1/1 -> Product_7a064/2
  State_iq_line_5_6_03d26/1 -> Product_4d4ad/2
  Product_7a064/1 -> Subtract_f6ff4/1
  Constant_2217.59481429868_1f2a1/1 -> Product_e5a10/1
  Product_4d4ad/1 -> Subtract_f6ff4/2
  Product_584f5/1 -> Subtract_6c7cf/2
  State_vq_bus_5_5a835/1 -> Product_e5a10/2
  Subtract_f6ff4/1 -> Add_0d293/1
  Product_e5a10/1 -> Add_0d293/2
  Constant_2217.59481429868_393ef/1 -> Product_584f5/1
  State_vq_bus_6_e6417/1 -> Product_584f5/2
  Add_0d293/1 -> Subtract_6c7cf/1

== system IEEE9Buses/AC_1/d_iq_line_6_7_block ==
  note: d_iq_line_6_7 in SG9
      | $3739.99125427356\,\mathrm{vq}_{\mathrm{bus},6}-44.5058959258554\,\mathrm{iq}_{\mathrm{line},6,7}-376.991118430775\,\mathrm{id}_{\mathrm{line},6,7}-3739.99125427356\,\mathrm{vq}_{\mathrm{bus},7}$
      | Automatically generated on 2025-09-12 21:34:40 .
  State_id_line_6_7_95748 : Inport
  State_iq_line_6_7_68911 : Inport  Port=2
  State_vq_bus_6_aeffa : Inport  Port=3
  State_vq_bus_7_cc662 : Inport  Port=4
  Add_62fe0 : Sum
  Constant_-376.991118430775_eeb63 : Constant  Value=-376.991118430775
  Constant_3739.99125427356_0d391 : Constant  Value=3739.99125427356
  Constant_3739.99125427356_e9f3f : Constant  Value=3739.99125427356
  Constant_44.5058959258554_29782 : Constant  Value=44.5058959258554
  Product_6866d : Product
  Product_783df : Product
  Product_a7854 : Product
  Product_fd086 : Product
  Subtract_b8d9f : Sum  Inputs=+-
  Subtract_d4168 : Sum  Inputs=+-
  Blockout_d_iq_line_6_7_a4a1a : Outport
  wires:
  Constant_-376.991118430775_eeb63/1 -> Product_783df/1
  Constant_44.5058959258554_29782/1 -> Product_fd086/1
  State_id_line_6_7_95748/1 -> Product_783df/2
  State_iq_line_6_7_68911/1 -> Product_fd086/2
  Product_783df/1 -> Subtract_b8d9f/1
  Constant_3739.99125427356_e9f3f/1 -> Product_a7854/1
  Product_fd086/1 -> Subtract_b8d9f/2
  State_vq_bus_6_aeffa/1 -> Product_a7854/2
  Subtract_b8d9f/1 -> Add_62fe0/1
  Product_a7854/1 -> Add_62fe0/2
  Constant_3739.99125427356_0d391/1 -> Product_6866d/1
  State_vq_bus_7_cc662/1 -> Product_6866d/2
  Add_62fe0/1 -> Subtract_d4168/1
  Product_6866d/1 -> Subtract_d4168/2
  Subtract_d4168/1 -> Blockout_d_iq_line_6_7_a4a1a/1

== system IEEE9Buses/AC_1/d_iq_line_7_8_block ==
  note: d_iq_line_7_8 in SG9
      | $5235.98775598299\,\mathrm{vq}_{\mathrm{bus},7}-44.5058959258554\,\mathrm{iq}_{\mathrm{line},7,8}-376.991118430775\,\mathrm{id}_{\mathrm{line},7,8}-5235.98775598299\,\mathrm{vq}_{\mathrm{bus},8}$
      | Automatically generated on 2025-09-12 21:34:42 .
  State_id_line_7_8_521a4 : Inport
  State_iq_line_7_8_5efa1 : Inport  Port=2
  State_vq_bus_7_5101f : Inport  Port=3
  State_vq_bus_8_ca51f : Inport  Port=4
  Add_6e6e0 : Sum
  Constant_-376.991118430775_8f361 : Constant  Value=-376.991118430775
  Constant_44.5058959258554_99a8c : Constant  Value=44.5058959258554
  Constant_5235.98775598299_0be36 : Constant  Value=5235.98775598299
  Constant_5235.98775598299_2c05d : Constant  Value=5235.98775598299
  Product_87734 : Product
  Product_d7860 : Product
  Product_dfe5b : Product
  Product_e8130 : Product
  Subtract_dab75 : Sum  Inputs=+-
  Subtract_f1efc : Sum  Inputs=+-
  Blockout_d_iq_line_7_8_47c62 : Outport
  wires:
  Constant_-376.991118430775_8f361/1 -> Product_d7860/1
  Constant_44.5058959258554_99a8c/1 -> Product_e8130/1
  State_id_line_7_8_521a4/1 -> Product_d7860/2
  State_iq_line_7_8_5efa1/1 -> Product_e8130/2
  Product_d7860/1 -> Subtract_dab75/1
  Constant_5235.98775598299_0be36/1 -> Product_dfe5b/1
  Product_e8130/1 -> Subtract_dab75/2
  State_vq_bus_7_5101f/1 -> Product_dfe5b/2
  Subtract_dab75/1 -> Add_6e6e0/1
  Product_dfe5b/1 -> Add_6e6e0/2
  Constant_5235.98775598299_2c05d/1 -> Product_87734/1
  State_vq_bus_8_ca51f/1 -> Product_87734/2
  Add_6e6e0/1 -> Subtract_f1efc/1
  Product_87734/1 -> Subtract_f1efc/2
  Subtract_f1efc/1 -> Blockout_d_iq_line_7_8_47c62/1

== system IEEE9Buses/AC_1/d_iq_line_8_2_block ==
  note: d_iq_line_8_2 in SG9
      | $6031.8578948924\,\mathrm{vq}_{\mathrm{bus},8}-6031.8578948924\,\mathrm{vq}_{\mathrm{bus},2}-376.991118430775\,\mathrm{id}_{\mathrm{line},8,2}$
      | Automatically generated on 2025-09-12 21:34:44 .
  State_id_line_8_2_1a8da : Inport
  State_vq_bus_2_6a8ad : Inport  Port=2
  State_vq_bus_8_54d3e : Inport  Port=3
  Add_e2ad1 : Sum
  Constant_-376.991118430775_9dbfa : Constant  Value=-376.991118430775
  Constant_6031.8578948924_58b70 : Constant  Value=6031.8578948924
  Constant_6031.8578948924_e3dd0 : Constant  Value=6031.8578948924
  Product_6ef32 : Product
  Product_ebe35 : Product
  Product_ec335 : Product
  Subtract_6dd02 : Sum  Inputs=+-
  Blockout_d_iq_line_8_2_3b9b1 : Outport
  wires:
  Constant_-376.991118430775_9dbfa/1 -> Product_6ef32/1
  Product_ebe35/1 -> Subtract_6dd02/2
  State_id_line_8_2_1a8da/1 -> Product_6ef32/2
  Constant_6031.8578948924_58b70/1 -> Product_ebe35/1
  Product_6ef32/1 -> Subtract_6dd02/1
  State_vq_bus_2_6a8ad/1 -> Product_ebe35/2
  Constant_6031.8578948924_e3dd0/1 -> Product_ec335/1
  State_vq_bus_8_54d3e/1 -> Product_ec335/2
  Subtract_6dd02/1 -> Add_e2ad1/1
  Product_ec335/1 -> Add_e2ad1/2
  Add_e2ad1/1 -> Blockout_d_iq_line_8_2_3b9b1/1

== system IEEE9Buses/AC_1/d_iq_line_8_9_block ==
  note: d_iq_line_8_9 in SG9
      | $2341.55974180606\,\mathrm{vq}_{\mathrm{bus},8}-74.9299117377938\,\mathrm{iq}_{\mathrm{line},8,9}-376.991118430775\,\mathrm{id}_{\mathrm{line},8,9}-2341.55974180606\,\mathrm{vq}_{\mathrm{bus},9}$
      | Automatically generated on 2025-09-12 21:34:46 .
  State_id_line_8_9_9ac4c : Inport
  State_iq_line_8_9_4d480 : Inport  Port=2
  State_vq_bus_8_a4521 : Inport  Port=3
  State_vq_bus_9_bbb4a : Inport  Port=4
  Add_804d7 : Sum
  Constant_-376.991118430775_338a8 : Constant  Value=-376.991118430775
  Constant_2341.55974180606_0d26e : Constant  Value=2341.55974180606
  Constant_2341.55974180606_d5295 : Constant  Value=2341.55974180606
  Constant_74.9299117377938_f15f6 : Constant  Value=74.9299117377938
  Product_485b3 : Product
  Product_57c85 : Product
  Product_7b998 : Product
  Product_9d4ca : Product
  Subtract_3f9db : Sum  Inputs=+-
  Subtract_a97f5 : Sum  Inputs=+-
  Blockout_d_iq_line_8_9_a326a : Outport
  wires:
  Constant_-376.991118430775_338a8/1 -> Product_485b3/1
  Constant_74.9299117377938_f15f6/1 -> Product_7b998/1
  State_id_line_8_9_9ac4c/1 -> Product_485b3/2
  State_iq_line_8_9_4d480/1 -> Product_7b998/2
  Product_485b3/1 -> Subtract_a97f5/1
  Constant_2341.55974180606_0d26e/1 -> Product_57c85/1
  Product_7b998/1 -> Subtract_a97f5/2
  State_vq_bus_8_a4521/1 -> Product_57c85/2
  Subtract_a97f5/1 -> Add_804d7/1
  Product_57c85/1 -> Add_804d7/2
  Constant_2341.55974180606_d5295/1 -> Product_9d4ca/1
  Add_804d7/1 -> Subtract_3f9db/1
  State_vq_bus_9_bbb4a/1 -> Product_9d4ca/2
  Product_9d4ca/1 -> Subtract_3f9db/2
  Subtract_3f9db/1 -> Blockout_d_iq_line_8_9_a326a/1

== system IEEE9Buses/AC_1/d_iq_line_9_4_block ==
  note: d_iq_line_9_4 in SG9
      | $4435.18962859735\,\mathrm{vq}_{\mathrm{bus},9}-44.3518962859735\,\mathrm{iq}_{\mathrm{line},9,4}-4435.18962859735\,\mathrm{vq}_{\mathrm{bus},4}-376.991118430775\,\mathrm{id}_{\mathrm{line},9,4}$
      | Automatically generated on 2025-09-12 21:34:48 .
  State_id_line_9_4_069c7 : Inport
  State_iq_line_9_4_5ae9b : Inport  Port=2
  State_vq_bus_4_81c39 : Inport  Port=3
  State_vq_bus_9_ae56d : Inport  Port=4
  Add_db2b5 : Sum
  Constant_-376.991118430775_4a099 : Constant  Value=-376.991118430775
  Constant_44.3518962859735_87876 : Constant  Value=44.3518962859735
  Constant_4435.18962859735_43734 : Constant  Value=4435.18962859735
  Constant_4435.18962859735_e7810 : Constant  Value=4435.18962859735
  Product_0afb7 : Product
  Product_14f5d : Product
  Product_b8917 : Product
  Product_e7ac2 : Product
  Subtract_6dde0 : Sum  Inputs=+-
  Subtract_9edf2 : Sum  Inputs=+-
  Blockout_d_iq_line_9_4_42bd3 : Outport
  wires:
  Constant_-376.991118430775_4a099/1 -> Product_14f5d/1
  Constant_44.3518962859735_87876/1 -> Product_0afb7/1
  State_id_line_9_4_069c7/1 -> Product_14f5d/2
  State_iq_line_9_4_5ae9b/1 -> Product_0afb7/2
  Product_14f5d/1 -> Subtract_6dde0/1
  Constant_4435.18962859735_43734/1 -> Product_b8917/1
  Product_0afb7/1 -> Subtract_6dde0/2
  State_vq_bus_4_81c39/1 -> Product_b8917/2
  Subtract_6dde0/1 -> Subtract_9edf2/1
  Product_b8917/1 -> Subtract_9edf2/2
  Constant_4435.18962859735_e7810/1 -> Product_e7ac2/1
  Add_db2b5/1 -> Blockout_d_iq_line_9_4_42bd3/1
  State_vq_bus_9_ae56d/1 -> Product_e7ac2/2
  Subtract_9edf2/1 -> Add_db2b5/1
  Product_e7ac2/1 -> Add_db2b5/2

== system IEEE9Buses/AC_1/d_iq_load_5_block ==
  note: d_iq_load_5 in SG9
      | $1188.5640696821\,\mathrm{vq}_{\mathrm{bus},5}-1130.97335529233\,\mathrm{iq}_{\mathrm{load},5}-376.991118430775\,\mathrm{id}_{\mathrm{load},5}$
      | Automatically generated on 2025-09-12 21:34:26 .
  State_id_load_5_3469a : Inport
  State_iq_load_5_30dc2 : Inport  Port=2
  State_vq_bus_5_8a47c : Inport  Port=3
  Add_138ff : Sum
  Constant_-376.991118430775_59aa5 : Constant  Value=-376.991118430775
  Constant_1130.97335529233_3ea9a : Constant  Value=1130.97335529233
  Constant_1188.5640696821_4893a : Constant  Value=1188.5640696821
  Product_78028 : Product
  Product_98e33 : Product
  Product_efe63 : Product
  Subtract_721c8 : Sum  Inputs=+-
  Blockout_d_iq_load_5_26519 : Outport
  wires:
  Constant_-376.991118430775_59aa5/1 -> Product_78028/1
  Product_efe63/1 -> Subtract_721c8/2
  State_id_load_5_3469a/1 -> Product_78028/2
  Constant_1130.97335529233_3ea9a/1 -> Product_efe63/1
  Product_78028/1 -> Subtract_721c8/1
  State_iq_load_5_30dc2/1 -> Product_efe63/2
  Constant_1188.5640696821_4893a/1 -> Product_98e33/1
  State_vq_bus_5_8a47c/1 -> Product_98e33/2
  Subtract_721c8/1 -> Add_138ff/1
  Product_98e33/1 -> Add_138ff/2
  Add_138ff/1 -> Blockout_d_iq_load_5_26519/1

== system IEEE9Buses/AC_1/d_iq_load_7_block ==
  note: d_iq_load_7 in SG9
      | $1244.53892235533\,\mathrm{vq}_{\mathrm{bus},7}-1077.11748123079\,\mathrm{iq}_{\mathrm{load},7}-376.991118430775\,\mathrm{id}_{\mathrm{load},7}$
      | Automatically generated on 2025-09-12 21:34:28 .
  State_id_load_7_27cc0 : Inport
  State_iq_load_7_db75c : Inport  Port=2
  State_vq_bus_7_44ad8 : Inport  Port=3
  Add_eec27 : Sum
  Constant_-376.991118430775_bac3b : Constant  Value=-376.991118430775
  Constant_1077.11748123079_58a41 : Constant  Value=1077.11748123079
  Constant_1244.53892235533_d908d : Constant  Value=1244.53892235533
  Product_88f50 : Product
  Product_8fef7 : Product
  Product_bd8e9 : Product
  Subtract_92dbf : Sum  Inputs=+-
  Blockout_d_iq_load_7_b1dc5 : Outport
  wires:
  Constant_-376.991118430775_bac3b/1 -> Product_8fef7/1
  Product_88f50/1 -> Subtract_92dbf/2
  State_id_load_7_27cc0/1 -> Product_8fef7/2
  Constant_1077.11748123079_58a41/1 -> Product_88f50/1
  Product_8fef7/1 -> Subtract_92dbf/1
  State_iq_load_7_db75c/1 -> Product_88f50/2
  Constant_1244.53892235533_d908d/1 -> Product_bd8e9/1
  State_vq_bus_7_44ad8/1 -> Product_bd8e9/2
  Subtract_92dbf/1 -> Add_eec27/1
  Product_bd8e9/1 -> Add_eec27/2
  Add_eec27/1 -> Blockout_d_iq_load_7_b1dc5/1

== system IEEE9Buses/AC_1/d_iq_load_9_block ==
  note: d_iq_load_9 in SG9
      | $1490.22474585066\,\mathrm{vq}_{\mathrm{bus},9}-942.477796076938\,\mathrm{iq}_{\mathrm{load},9}-376.991118430775\,\mathrm{id}_{\mathrm{load},9}$
      | Automatically generated on 2025-09-12 21:34:29 .
  State_id_load_9_2692c : Inport
  State_iq_load_9_d6a72 : Inport  Port=2
  State_vq_bus_9_5d2b3 : Inport  Port=3
  Add_16b5e : Sum
  Constant_-376.991118430775_a4dee : Constant  Value=-376.991118430775
  Constant_1490.22474585066_5d063 : Constant  Value=1490.22474585066
  Constant_942.477796076938_12444 : Constant  Value=942.477796076938
  Product_2505a : Product
  Product_5ca35 : Product
  Product_e7c20 : Product
  Subtract_d2985 : Sum  Inputs=+-
  Blockout_d_iq_load_9_040c9 : Outport
  wires:
  Constant_-376.991118430775_a4dee/1 -> Product_e7c20/1
  Product_5ca35/1 -> Subtract_d2985/2
  State_id_load_9_2692c/1 -> Product_e7c20/2
  Add_16b5e/1 -> Blockout_d_iq_load_9_040c9/1
  Constant_942.477796076938_12444/1 -> Product_5ca35/1
  Product_2505a/1 -> Add_16b5e/2
  Product_e7c20/1 -> Subtract_d2985/1
  State_iq_load_9_d6a72/1 -> Product_5ca35/2
  Constant_1490.22474585066_5d063/1 -> Product_2505a/1
  State_vq_bus_9_5d2b3/1 -> Product_2505a/2
  Subtract_d2985/1 -> Add_16b5e/1

== system IEEE9Buses/AC_1/d_vd_bus_1_block ==
  note: d_vd_bus_1 in SG9
      | $37699111.8430775\,\mathrm{id}_{\mathrm{bus},1}+376.991118430775\,\mathrm{vq}_{\mathrm{bus},1}$
      | Automatically generated on 2025-09-12 21:34:11 .
  Alge_id_bus_1_5efe2 : Inport
  State_vq_bus_1_fa40c : Inport  Port=2
  Add_adff1 : Sum
  Constant_376.991118430775_a930f : Constant  Value=376.991118430775
  Constant_37699111.8430775_a186f : Constant  Value=37699111.8430775
  Product_af6b4 : Product
  Product_f5d81 : Product
  Blockout_d_vd_bus_1_31f38 : Outport
  wires:
  Constant_37699111.8430775_a186f/1 -> Product_af6b4/1
  Product_f5d81/1 -> Add_adff1/2
  Alge_id_bus_1_5efe2/1 -> Product_af6b4/2
  Constant_376.991118430775_a930f/1 -> Product_f5d81/1
  State_vq_bus_1_fa40c/1 -> Product_f5d81/2
  Add_adff1/1 -> Blockout_d_vd_bus_1_31f38/1
  Product_af6b4/1 -> Add_adff1/1
